simulink model "may14bdrc"  (R2015a)
settings: Solver=ode4  StartTime=0.0  StopTime=inf  FixedStep=BKIN_STEP_TIME  RelTol=1e-3
StartFcn:
  |  warndlg('Dexterit-E models cannot run under simulation. Please compile your model and run it from within Dexterit-E.');set_param(bdroot,'SimulationCommand','stop')
model workspace (MAT data in the model file):
  BARRIER_ROW = 5
  BKIN_KINEMATIC_FRAME_SIZE = 400
  BKIN_STEP_TIME = 0.00025
  CIRCLE_ROW = 2
  CIRCLE_STROKE = 10
  CIRCLE_STROKE_W = 11
  E_BARRIER_HIT = 6
  E_COLLISION_HIT = 7
  E_ENTER_PRESHOT_AREA = 2
  E_ENTER_START_AREA = 12
  E_EXIT = 13
  E_EXIT_PRESHOT_AREA = 10
  E_GOAL_HIT = 8
  E_GOAL_REACHED = 5
  E_NO_EVENT = 0
  E_PRESHOT_ROW = 4
  E_TARGET_OUT_OF_BOUNDS = 9
  E_TRIAL_BEGIN = 1
  E_TRIAL_ENDED = 3
  FIRST_STATE_FILL = 9
  FORCE_MULTIPLIER = 1
  F_BUMP = 1
  GOAL_ROW = 8
  GOAL_TIME = 15
  HEIGHT = 6
  INVISIBLE_FILL = 15
  LOAD_ROW = 4
  MASS_BARRIER = 6
  MASS_CIRCLE = 2
  MASS_RECT = 3
  NEW_FLOAT = 10
  NEW_ROW = 9
  NEW_TEXTSIZE = 11
  PERT_DUR = 5
  PERT_RAMP = 4
  PRESHOT_ROW = 7
  RADIUS_LOG = 4
  RADIUS_VIS = 5
  RECT_FILL = 12
  RECT_ROW = 3
  RECT_STROKE = 13
  RECT_STROKE_W = 14
  ROTATION = 7
  SECONDS = 1
  SECOND_STATE_FILL = 8
  SHOT_READY_TIME = 13
  SHOT_SET_TIME = 14
  START_HOLD_TIME = 12
  START_ROW = 6
  TRIAL_FAILURE = 11
  WIDTH = 3
  col_x = 1
  col_y = 2
undefined symbols (not defined in the file): slselsubs
libraries: Video x7, General x3, KINARM_loads x2, KINARM_EP_loads x1, KINARM_general x1, simulink x1, slrtlib x1
(part 2 of 3)

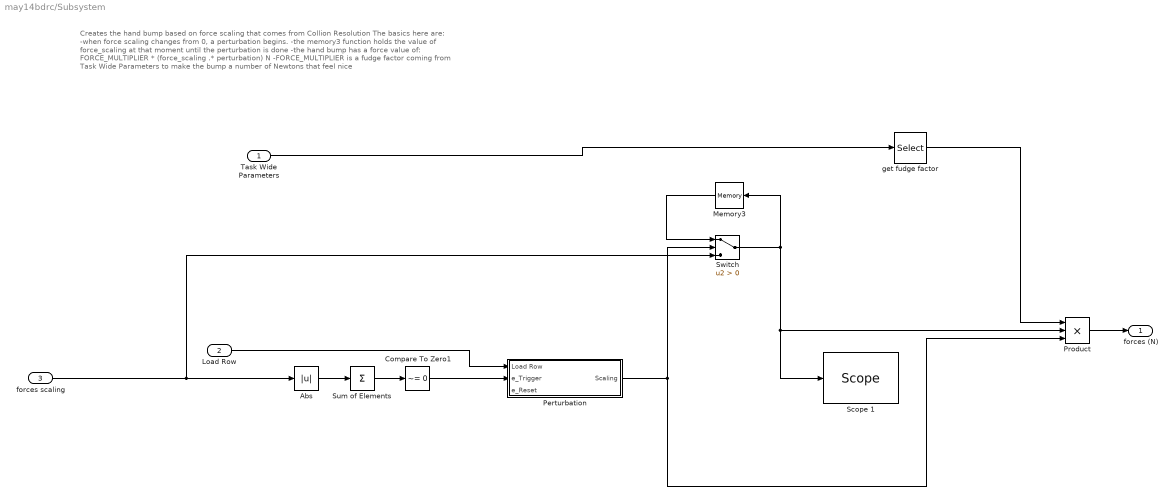
== system may14bdrc/Subsystem ==
  note: Creates the hand bump based on force scaling that comes from Collion Resolution
      |
      | The basics here are:
      | -when force scaling changes from 0, a perturbation begins.
      | -the memory3 function holds the value of force_scaling at that moment until the perturbation is done
      | -the hand bump has a force value of: FORCE_MULTIPLIER * (force_scaling .* perturbation) N
      | -FORCE_MULTIPLIER is a fudge factor coming from Task Wide Parameters to make the bump a number of Newtons that feel nice
  Task Wide Parameters : Inport
  Load Row : Inport  Port=2
  forces scaling : Inport  Port=3
  Abs : Abs
  Compare To Zero1 : simulink/Logic and Bit Operations/Compare To Zero  relop=~=  OutDataTypeStr=uint8  ZeroCross=off
  Memory3 : Memory  InheritSampleTime=on
  Perturbation : Subsystem  AncestorBlock=KINARM_loads/Perturbation  mask(Perturbation){loadcol=[PERT_RAMP PERT_DUR PERT_RAMP]}
      mask prompts: loadcol "Load Table Columns [colA colB colC]"
      mask help:
      | The Perturbation block creates a time-varying output that is used to ‘window’ the output of other load  blocks.  For example, to create a force pulse, the 'scaling' output of this block would be wired into the 'scaling' input of the Constant_Loads_(hand) block.
      |
      | The shape of the scaling window is trapezoidal and composed of three sections:
      |
      | 1. A linear on-ramp where the scaling output goes from 0 to 1. The duration of this ramping is determined from the value in column A.
      | 2. A duration where the scaling output is 1 (i.e. maximal). This duration is determined from the value in column B.
      | 3. A linear off-ramp where the scaling output goes from 1 to 0. The duration of this ramping is determined from the value in column C.
      |
      | (Note: scaling output = 0 between perturbations)
      |
      | The values in columns A, B & C must all be in milliseconds.
      |
      | The reset input is used to immediately stop the perturbation and set the output scaling to zero. The reset input does not need to be called between uses.
      mask init:
      | library = 'KINARM_loads';
      | numCol = 3;
      | [inputname1, inputname2, inputname3, outputname, columntext] = loadBlockInitCommands(gcb, library, numCol);
      mask Help:
      | Used to create a perturbation 'window' for scaling other load blocks.
      | 
      | <H2>Library </H2>
      | KINARM EXO loads
      | 
      | <H2>Description </H2>
      | The Perturbation block creates a time-varying output that is used to ‘window’ the output of other load blocks.  The 'scaling' output of the Perturbation block is typically wired to the 'scaling' input of another load block (note: the 'scaling' input of other loads blocks is hidden by default and must be shown by setting the 'Source for scaling' to 'external' within that block’s dialog box).
      | <P>
      | <P>
      | The perturbation window is started by sending a Stateflow event to the trigger input.  Once the perturbation has started, it continues in a deterministic fashion to its end unless a Stateflow event is sent to the 'reset' input, in which case the perturbation is canceled and the 'scaling' output is set to 0.
      | 
      | <p>The shape of the scaling window is trapezoidal and composed of three sections:
      | 
      | <ol>
      | <li>A linear on-ramp where the scaling output goes from 0 to 1. The duration of this ramping is determined from the value in column A.</li>
      | <li>A duration where the scaling output is 1 (i.e. maximal). This duration is determined from the value in column B.</li>
      | <li>A linear off-ramp where the scaling output goes from 1 to 0. The duration of this ramping is determined from the value in column C.</li>
      | </ol>
      | 
      | The ramp duration parameters [A, B, C] are found in the Load Table using the 'row' input to this block and the 'columns' parameter found in the dialog box for this block.
      | <p>For example, if the "row" input = 2, and "Load Table columns" are specified as [1 2 3], then using the sample Load Table below, the duration of the on ramp is 100 ms, constant torque is 200 ms, and the off ramp is 500 ms.
      | <br>
      | (Note: scaling output = 0 between perturbations)
      | 
      | <table border="1" cellpadding="5">
      | <tr><td></td><td>Ramp On</td><td>Const</td><td>Ramp off</td></tr>
      | <tr><td>Load 1</td><td>25</td><td>25</td><td>25</td></tr>
      | <tr><td>Load 2</td><td>100</td><td>200</td><td>500</td></tr>
      | <tr><td>Load 3</td><td>25</td><td>50</td><td>75</td></tr>
      | </table>
      | <P>
      | <B>row: </B> this scalar input indicates which row in the Load Table the ramp duration parameters [A, B, C] will come from.
      | <P>
      | <B>trigger: </B> this Stateflow event input starts the perturbation (triggered on either rising or falling; the Stateflow output event providing this trigger should have its Trigger setting set to ‘either’).  This input will be ignored if the Perturbation block is presently executing a perturbation.
      | <P>
      | <B>reset: </B> this Stateflow event input resets the perturbation (triggered on either rising or falling).  The reset will act immediately and force the Scaling output =0. This does not need to be called between used of the block. If you do not need to stop a perturbation prematurely, then this input can remain unconnected.
      | <P>
      | <B>scaling: </B> this scalar output is the time-dependent window created by this block.  Typically it is wired to the 'scaling' input of another load block.  It ranges in value from 0 to 1.
      | 
      | <H2>Parameters and Dialog Box</H2>
      | <B>Load Table Columns:</B> a 3x1 vector with the elements corresponding to the columns in the Load Table for parameters A, B and C.  If a parameter is not going to be in the Load Table, then the value 0 should be used in the "Load Table Columns" vector (e.g. if there is to be no on-ramp or off-ramp, and the peak-duration coefficients is in column 2, then the "Load Table Columns" vector should be [0 2 0], which indicates that A and C are not specified in the Load Table and so they are set =0).  The same column may be used for more than one parameter, so if the on-ramp and off-ramp are to be equal, then the same column can be specified twice (e.g. [1 2 1]).
      | <P>
      |  All durations are specified in milliseconds.
      | 
      | <H2>Examples</H2>
      | <B>Example 1. </B> Suppose we wish to create a torque pulse with no on or off ramp and a peak duration specified in column 3 of the Load Table.  The 'scaling' output of the Perturbation block would be wired to the 'scaling' input of the Constant_Loads_(joints) block (after setting 'Source for scaling' to 'external' within the Constant_Loads_(joints) block).  The Load Table Columns setting in the dialog box for the Perturbation block would be set to [0 3 0], which indicates no on-ramp or off-ramp and that the peak duration will be in column 3 of the Load Table.
      | <P>
      | <B>Example 2. </B> Suppose we wish to create a force pulse at the hand with an on-ramp and off-ramp of the same duration (specified in column3 of the Load Table) and a peak duration specified in column 4 of the Load Table.  The 'scaling' output of the Perturbation block would be wired to the 'scaling' input of the Constant_Loads_(hand) block (after setting 'Source for scaling' to 'external' within the Constant_Loads_(hand) block).  The Load Table Columns setting in the dialog box for the Perturbation block would be set to [3 4 3], which indicates that the on-ramp and off-ramp durations are specified in column 3 of the Load Table and that the peak duration will be in column 4 of the Load Table.
      | 
      | <H2>Related Blocks </H2>
      | KINARM_Exo_Apply_Loads<BR>
      | Constant_Loads_(hand)<BR>
      | Constant_Loads_(joint)
      mask Callback loadcol:
      | %%%%
      | % Because of bugs iN R2007, R2010a and R2013a (which have been reported to Mathworks), the following code
      | % is required here because in the Initialization Section it will ONLY correctly update those Mask Parameters that are hidden
      | % when the OK button is clicked (NOTE: the initialization code will correctly update all Mask Parameters when the Apply button
      | % is clicked, the bug is that it should also update everything when the OK button is clicked in the absence of an Apply click)
      | %
      | % Adding a set_param call which updates one of the mask parameters will call the initialization code to run, which "avoids"
      | % this bug. This code should be removed once Mathworks has fixed this bug.
      | 
      | temp = get_param(gcb, 'loadcol');
      | set_param(gcb, 'loadcol', temp);
      mask Display:
      | disp(columntext);
      | port_label('output',1,outputname);
      | port_label('input',1, inputname1);
      | port_label('input',2, inputname2);
      | port_label('input',3, inputname3);
  Product : Product  Inputs=3
  Scope 1 : slrtlib/Displays and Logging/Scope   scopeno=4  scopetype=Target  autostart=off  viewmode=Graphical redraw  formatstr='%15.6f'  grid=on  ylimits=[0,0]  nosamples=250  noprepostsamples=0  interleave=1  triggermode=FreeRun  triggersignal=1  trigsignalfromport=off  triggerlevel=0.0  triggerslope=Either  triggerscope=1  triggersample=0  filename=data.dat  mode=Lazy  writesize=512  autorestart=off  dynamicfilemode=off  maxwritefilesize=512*1024^2
  Sum of Elements : Sum  Inputs=+
  Switch : Switch  Criteria=u2 > Threshold
  get fudge factor : Selector  IndexOptions=Index vector (dialog)  Indices=FORCE_MULTIPLIER  OutputSizes=1
  forces (N) : Outport
  wires:
  Compare To Zero1/1 -> Perturbation/2(e_Trigger)
  Sum of Elements/1 -> Compare To Zero1/1
  forces scaling/1 -> Switch/3, Abs/1
  get fudge factor/1 -> Product/1
  Switch/1 -> Memory3/1, Scope 1/1, Product/2
  Perturbation/1(Scaling) -> Product/3, Switch/2
  Abs/1 -> Sum of Elements/1
  Memory3/1 -> Switch/1
  Load Row/1 -> Perturbation/1(Load Row)
  Product/1 -> forces (N)/1
  Task Wide Parameters/1 -> get fudge factor/1

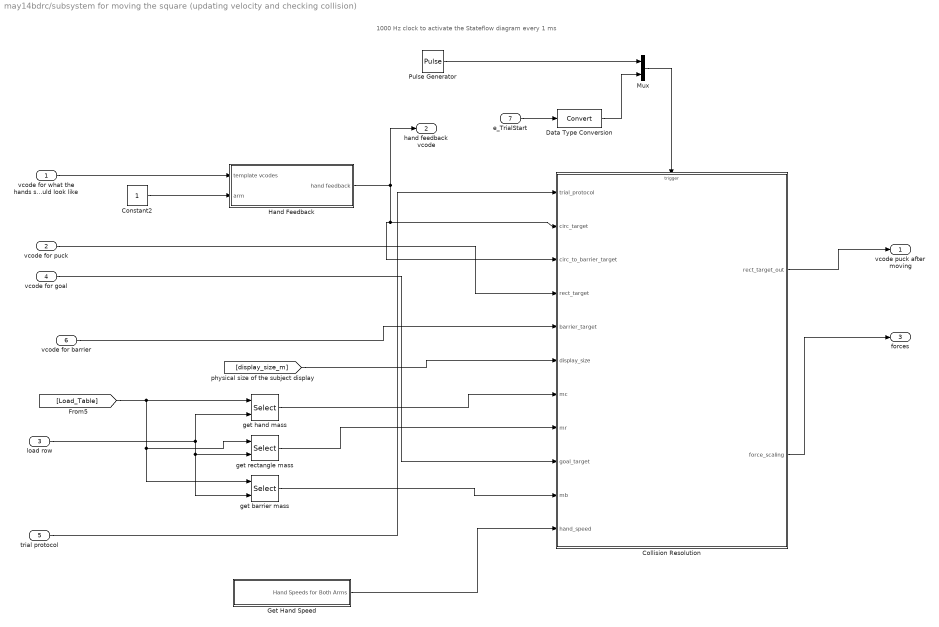
== system may14bdrc/subsystem for moving the square (updating velocity and checking collision) ==
  note: 1000 Hz clock to activate the Stateflow diagram every 1 ms
  vcode for what the hands should look like : Inport  PortDimensions=[1 70]
  vcode for puck : Inport  Port=2  PortDimensions=[1 70]  LockScale=on
  load row : Inport  Port=3
  vcode for goal : Inport  Port=4  PortDimensions=[1 70]
  trial protocol : Inport  Port=5
  vcode for barrier : Inport  Port=6  PortDimensions=[1 70]
  e_TrialStart : Inport  Port=7
  Collision Resolution : Stateflow chart  TreatAsAtomicUnit=on
      settings: PermitHierarchicalResolution=ParametersOnly
  Constant2 : Constant
  Data Type Conversion : DataTypeConversion
  Get Hand Speed : Subsystem
  Hand Feedback : Subsystem
  Mux : Mux  Inputs=2
  Pulse Generator : DiscretePulseGenerator  PulseType=Time based  Period=1/1000  PulseWidth=50
  get barrier mass : Selector  NumberOfDimensions=2  IndexOptions=Index vector (port),Index vector (dialog)  Indices=MASS_RECT,MASS_RECT  OutputSizes=1,1
  get hand mass : Selector  NumberOfDimensions=2  IndexOptions=Index vector (port),Index vector (dialog)  Indices=MASS_CIRCLE,MASS_CIRCLE  OutputSizes=1,1
  get rectangle mass : Selector  NumberOfDimensions=2  IndexOptions=Index vector (port),Index vector (dialog)  Indices=MASS_RECT,MASS_RECT  OutputSizes=1,1
  vcode puck after moving : Outport
  hand feedback vcode : Outport  Port=2
  forces : Outport  Port=3
  wires:
  load row/1 -> get barrier mass/2, get rectangle mass/2, get hand mass/2
  Hand Feedback/1(hand feedback) -> hand feedback vcode/1, Collision Resolution/3(circ_to_barrier_target), Collision Resolution/2(circ_target)
  Collision Resolution/1(rect_target_out) -> vcode puck after moving/1
  vcode for puck/1 -> Collision Resolution/4(rect_target)
  Get Hand Speed/1(Hand Speeds for Both Arms) -> Collision Resolution/11(hand_speed)
  get hand mass/1 -> Collision Resolution/7(mc)
  get rectangle mass/1 -> Collision Resolution/8(mr)
  Pulse Generator/1 -> Mux/1
  [display_size_m] -> Collision Resolution/6(display_size)
  Collision Resolution/2(force_scaling) -> forces/1
  vcode for what the hands should look like/1 -> Hand Feedback/1(template vcodes)
  Constant2/1 -> Hand Feedback/2(arm)
  vcode for goal/1 -> Collision Resolution/9(goal_target)
  trial protocol/1 -> Collision Resolution/1(trial_protocol)
  vcode for barrier/1 -> Collision Resolution/5(barrier_target)
  [Load_Table] -> get barrier mass/1, get rectangle mass/1, get hand mass/1
  get barrier mass/1 -> Collision Resolution/10(mb)
  Mux/1 -> Collision Resolution/Trigger
  e_TrialStart/1 -> Data Type Conversion/1
  Data Type Conversion/1 -> Mux/2

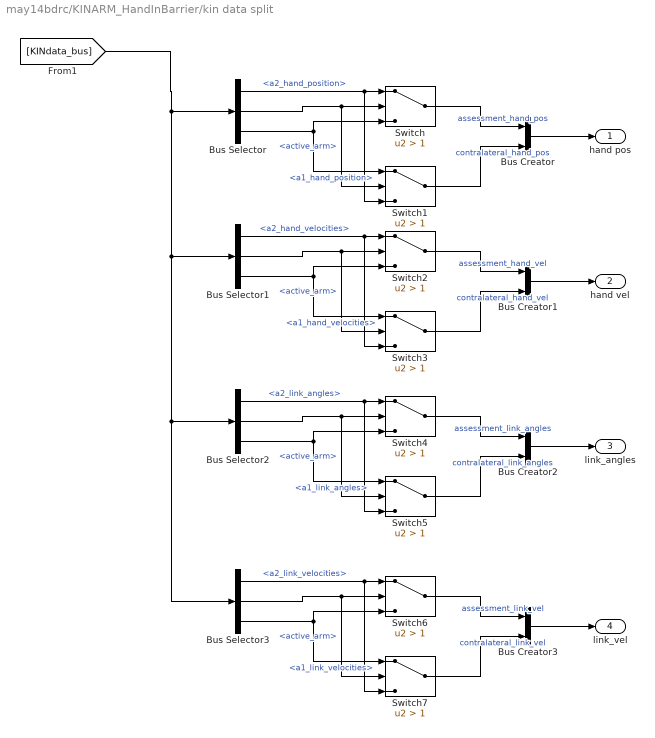
== system may14bdrc/KINARM_HandInBarrier/kin data split ==
  Bus Creator{,1..3} (4 alike) : BusCreator  Inputs=2
  Bus Selector : BusSelector  OutputSignals=Robot2.a2_hand_position,KINDataGeneral.active_arm,Robot1.a1_hand_position
  Bus Selector1 : BusSelector  OutputSignals=Robot2.a2_hand_velocities,KINDataGeneral.active_arm,Robot1.a1_hand_velocities
  Bus Selector2 : BusSelector  OutputSignals=Robot2.a2_link_angles,KINDataGeneral.active_arm,Robot1.a1_link_angles
  Bus Selector3 : BusSelector  OutputSignals=Robot2.a2_link_velocities,KINDataGeneral.active_arm,Robot1.a1_link_velocities
  Switch{,1..7} (8 alike) : Switch  Criteria=u2 > Threshold  Threshold=1
  hand pos : Outport
  hand vel : Outport  Port=2
  link_angles : Outport  Port=3
  link_vel : Outport  Port=4
  wires:
  Bus Selector/1 -> Switch1/3, Switch/1  "<a2_hand_position>"
  Switch/1 -> Bus Creator/1  "assessment_hand_pos"
  Switch1/1 -> Bus Creator/2  "contralateral_hand_pos"
  Bus Creator/1 -> hand pos/1
  Bus Selector/3 -> Switch1/1, Switch/3  "<a1_hand_position>"
  Bus Selector/2 -> Switch1/2, Switch/2  "<active_arm>"
  Bus Selector1/1 -> Switch3/3, Switch2/1  "<a2_hand_velocities>"
  Switch2/1 -> Bus Creator1/1  "assessment_hand_vel"
  Switch3/1 -> Bus Creator1/2  "contralateral_hand_vel"
  Bus Creator1/1 -> hand vel/1
  Bus Selector1/3 -> Switch3/1, Switch2/3  "<a1_hand_velocities>"
  Bus Selector1/2 -> Switch3/2, Switch2/2  "<active_arm>"
  Bus Selector2/1 -> Switch5/3, Switch4/1  "<a2_link_angles>"
  Switch4/1 -> Bus Creator2/1  "assessment_link_angles"
  Switch5/1 -> Bus Creator2/2  "contralateral_link_angles"
  Bus Creator2/1 -> link_angles/1
  Bus Selector2/3 -> Switch5/1, Switch4/3  "<a1_link_angles>"
  Bus Selector2/2 -> Switch5/2, Switch4/2  "<active_arm>"
  Bus Selector3/1 -> Switch7/3, Switch6/1  "<a2_link_velocities>"
  Switch6/1 -> Bus Creator3/1  "assessment_link_vel"
  Switch7/1 -> Bus Creator3/2  "contralateral_link_vel"
  Bus Creator3/1 -> link_vel/1
  [KINdata_bus] -> Bus Selector3/1, Bus Selector2/1, Bus Selector1/1, Bus Selector/1
  Bus Selector3/3 -> Switch7/1, Switch6/3  "<a1_link_velocities>"
  Bus Selector3/2 -> Switch7/2, Switch6/2  "<active_arm>"

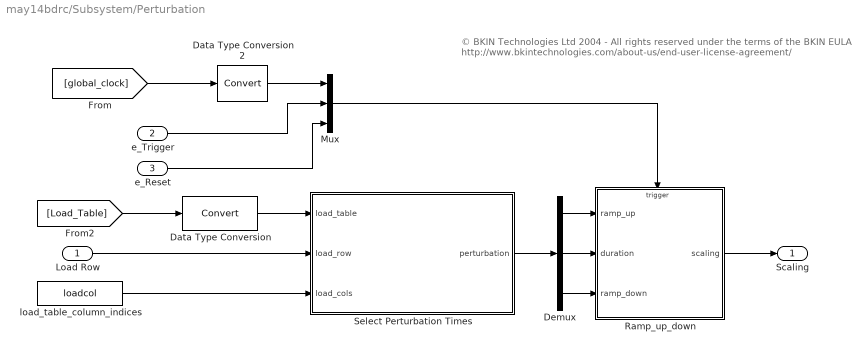
== system may14bdrc/Subsystem/Perturbation ==
  note: © BKIN Technologies Ltd 2004  - All rights reserved under the terms of the BKIN EULA
      | http://www.bkintechnologies.com/about-us/end-user-license-agreement/
  Load Row : Inport
  e_Trigger : Inport  Port=2
  e_Reset : Inport  Port=3
  Data Type Conversion : DataTypeConversion
  Data Type Conversion2 : DataTypeConversion
  Demux : Demux  Outputs=3
  Mux : Mux  Inputs=3
  Ramp_up_down : Stateflow chart  TreatAsAtomicUnit=on
      settings: PermitHierarchicalResolution=ParametersOnly
  Select Perturbation Times : MATLAB Function  TreatAsAtomicUnit=on
      settings: PermitHierarchicalResolution=ParametersOnly
  load_table_column_indices : Constant  Value=loadcol
  Scaling : Outport
  wires:
  Data Type Conversion2/1 -> Mux/1
  Mux/1 -> Ramp_up_down/Trigger
  Demux/3 -> Ramp_up_down/3(ramp_down)
  Demux/2 -> Ramp_up_down/2(duration)
  Demux/1 -> Ramp_up_down/1(ramp_up)
  [global_clock] -> Data Type Conversion2/1
  Ramp_up_down/1(scaling) -> Scaling/1
  e_Trigger/1 -> Mux/2
  e_Reset/1 -> Mux/3
  [Load_Table] -> Data Type Conversion/1
  Load Row/1 -> Select Perturbation Times/2(load_row)
  load_table_column_indices/1 -> Select Perturbation Times/3(load_cols)
  Select Perturbation Times/1(perturbation) -> Demux/1
  Data Type Conversion/1 -> Select Perturbation Times/1(load_table)

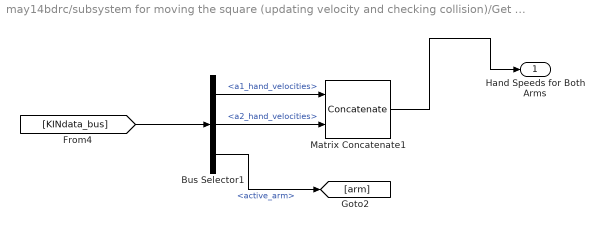
== system may14bdrc/subsystem for moving the square (updating velocity and checking collision)/Get Hand Speed ==
  Bus Selector1 : BusSelector  OutputSignals=Robot1.a1_hand_velocities,Robot2.a2_hand_velocities,KINDataGeneral.active_arm
  Matrix Concatenate1 : Concatenate  Mode=Multidimensional array
  Hand Speeds for Both Arms : Outport
  wires:
  [KINdata_bus] -> Bus Selector1/1
  Bus Selector1/1 -> Matrix Concatenate1/1  "<a1_hand_velocities>"
  Matrix Concatenate1/1 -> Hand Speeds for Both Arms/1
  Bus Selector1/2 -> Matrix Concatenate1/2  "<a2_hand_velocities>"
  Bus Selector1/3 -> [arm]  "<active_arm>"

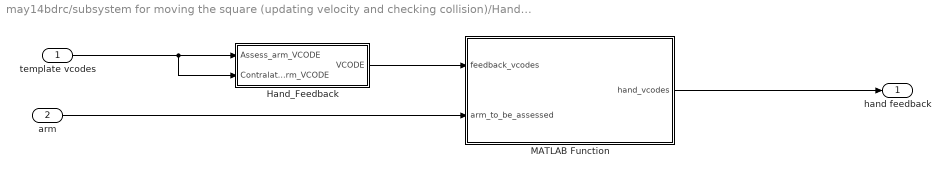
== system may14bdrc/subsystem for moving the square (updating velocity and checking collision)/Hand Feedback ==
  template vcodes : Inport
  arm : Inport  Port=2
  Hand_Feedback : Subsystem  AncestorBlock=KINARM_general/Hand_Feedback  mask(Hand_Feedback){feedback_cntl_src=style and status}
      mask prompts: feedback_cntl_src "Task Program control of style and status"
      mask help:
      | This block controls various options for hand feedback (i.e. fingertip position)  to be shown to the subject.
      |
      | Task Program control of style and status refers to whether the Program Task will explicity control the style and/or status of the hand feedback.
      mask init:
      | block_path = gcb;  % store block path, as gcb may change with block operations
      | 
      | %%% Handle background colours if link status changes.  
      | checkBackgroundColour(block_path, 'KINARM_general');
      | 
      | 
      | feedback_cntl_source=get_param(gcb,'feedback_cntl_src');
      | 
      | if feedback_cntl_source(1:4)=='none'
      |     block1type='Constant';
      |     block2type='Constant';
      |     block3type='Constant';
      | elseif feedback_cntl_source(1:4)=='stat'
      |     block1type='Constant';
      |     block2type='Constant';
      |     block3type='Inport';
      | else 
      |     block1type='Inport';
      |     block2type='Inport';
      |     block3type='Constant';
      | end
      | 
      | hasOldName1 = ~isempty(find_system(gcb, 'FollowLinks', 'on', 'LookUnderMasks', 'all', 'name', 'Dom_VCODE'));
      | hasOldName2 = ~isempty(find_system(gcb, 'FollowLinks', 'on', 'LookUnderMasks', 'all', 'name', 'non-Dom_VCODE'));
      | 
      | block1name='Assess_arm_VCODE';
      | block2name='Contralateral_arm_VCODE';
      | block1path=[gcb '/' block1name];
      | block2path=[gcb '/' block2name];
      | 
      | if hasOldName1
      | 	set_param([gcb '/Dom_VCODE'],'name', block1name);
      | end
      | 
      | if hasOldName2
      | 	set_param([gcb '/non-Dom_VCODE'],'name', block2name);
      | end
      | 
      | if ~strcmp(get_param(block1path,'blocktype'),block1type)
      | 	pos=get_param(block1path,'position');
      | 	delete_line(gcb, [block1name '/1'], 'Reshape/1');
      | 	delete_block(block1path);
      | 	add_block(['built-in/' block1type], block1path,'Name',block1name);
      | 	set_param(block1path,'position',pos);
      | 	add_line(gcb, [block1name '/1'], 'Reshape/1');
      | end
      | 
      | if ~strcmp(get_param(block2path,'blocktype'),block2type)
      | 	pos=get_param(block2path,'position');
      | 	delete_line(gcb, [block2name '/1'], 'Reshape1/1');
      | 	delete_block(block2path);
      | 	add_block(['built-in/' block2type],block2path,'Name',block2name);
      | 	set_param(block2path,'position',pos);
      | 	add_line(gcb, [block2name '/1'], 'Reshape1/1');
      | end
      | 
      | block3name='feedback_status';
      | block3path=[gcb '/' block3name];
      | if ~strcmp(get_param(block3path,'blocktype'),block3type)
      | 	pos=get_param(block3path,'position');
      | 	delete_line(gcb, [block3name '/1'], 'FeedFwdArm/3');
      | 	delete_block(block3path);
      | 	add_block(['built-in/' block3type],block3path,'Name',block3name);
      | 	set_param(block3path,'position',pos);
      | 	add_line(gcb, [block3name '/1'], 'FeedFwdArm/3');
      | end
      | 
      | if feedback_cntl_source(1:4)=='none'
      | 	set_param(block1path,'Value','[1:70]');
      | 	set_param(block2path,'Value','[71:140]');
      | elseif feedback_cntl_source(1:4)=='stat'
      | 	set_param(block1path,'Value','[1:70]');
      | 	set_param(block2path,'Value','[71:140]');
      | end
      mask Help:
      | Creates VCODE for drawing hand position (fingertip).
      | <P>
      | <H2>Library </H2>
      | KINARM general
      | 
      | <H2>Description </H2>
      | This block controls various options for drawing hand feedback.  (Note: although it is called hand feedback, it is actually the fingertip position that is shown).  Three options are available (as chosen in the Parameters and Dialog box):
      | <P>
      | (i) GUI control of feedback style and status
      | <Blockquote>
      | No inputs are required for this option.  The Task Program has no control over the style or status of the hand feedback.
      | </Blockquote>
      | (ii) Task Program control of feedback status and GUI control of style
      | <Blockquote>
      | If Task Program control of feedback status is chosen, then one input appears for this block:<P>
      | <B> feedback_status: </B> this scalar input dynamically controls the status of the hand feedback as per the following:
      | <P>
      | 0 = (no hand feedback)<BR>
      | 1 = ("arm to be assessed" hand feedback only)<BR>
      | 2 = (contralateral arm hand feedback only)<BR>
      | 3 = (hand feedback on for both hands)<BR>
      | </Blockquote>
      | (iii) Task Program control of both feedback style and status.
      | <Blockquote>
      | 
      | If Task Program control of feedback status and style is chosen, then two inputs appear for this block:<P>
      | <B> Assess_arm_VCODE: </B>  this vector input dynamically controls the status and style of the hand feedback for the "arm to be assessed" the operator selected in Dexterit-E.
      | <P>
      | <B> Contralateral_arm_VCODE:</B>  this vector input dynamically controls the status and style of the hand feedback for the contralateral hand.
      | <P>
      | For both the Assess_arm_VCODE and the Contralateral_arm_VCODE, the input vectors must be in the appropriate VCODE format (for more information on the details of a VCODE, please right click on the Show_Target block in the video library, "Look Under Mask" and open the Embedded Matlab function).  Note that the position information in the Dom_VCODE and non-Dom_VCODE are overwritten in this block, but all other aspects of the VCODE are passed through to the output.
      | </Blockquote>
      | Note that if Task Program control is chosen for either hand feedback status or style, the GUI will still override these settings if the Task Protocol specifies that it should do so.
      | <P>
      | There is one output from this block:
      | <P>
      | <B> VCODE: </B> this output is 2-row matrix containing 2 VCODEs.  The first VCODE is for the dominant hand feedback and the second VCODE is for the non-dominant hand feedback.  This output must go to the Process_Video_CMD block of the video library for the hand feedback to actually be shown (if any other visual targets are to be displayed, then this VCODE output must be concatenated with the other VCODES prior to connection to the Process_Video_CMD block - see Help for the Process_Video_CMD block for more information).
      | <H2>Parameters and Dialog Box</H2>
      | <B>Task Program control of style and status</B> refers to whether the Program Task will explicity control the style and/or status of the hand feedback.  The three options are: none, status only, or status and style.
      | <P>
      |  - Choosing none means that style and status are always controlled by the GUI.
      | <P>
      |  - Choosing status only means that the GUI always controls the hand feedback style, but also will create an input to this block allowing the end user to control the status dynamically.  Allowable input values are: 0 (no hand feedback), 1 (dominant hand feedback only), 2 (non-dominant hand feedback only) or 3 (hand feedback on for both hands)
      |  <P>
      | - Choosing status and style means that both the hand feedback status and style can be controlled dynamically by the Task Program.  If this option is selected, then two inputs will be created for this block: dominant VCODE and non-dominant VCODE.  These two inputs require a proper VCODE (e.g. from a Show_Target block) for each.  Because status and style are both part of a VCODE, there is no separate input for hand feedback status.  Note: any position information of these input VCODEs is overwritten by this block by the appropriate fingertip locations.
      | <P>
      | 
      | <H2>Related Blocks </H2>
      | DataLogging<BR>
      | Show_Target<BR>
      | Process_Video_CMD
      mask TypeOptions feedback_cntl_src: none | status only | style and status
  MATLAB Function : MATLAB Function  TreatAsAtomicUnit=on
      settings: PermitHierarchicalResolution=ParametersOnly
  hand feedback : Outport
  wires:
  template vcodes/1 -> Hand_Feedback/2(Contralateral_arm_VCODE), Hand_Feedback/1(Assess_arm_VCODE)
  Hand_Feedback/1(VCODE) -> MATLAB Function/1(feedback_vcodes)
  arm/1 -> MATLAB Function/2(arm_to_be_assessed)
  MATLAB Function/1(hand_vcodes) -> hand feedback/1

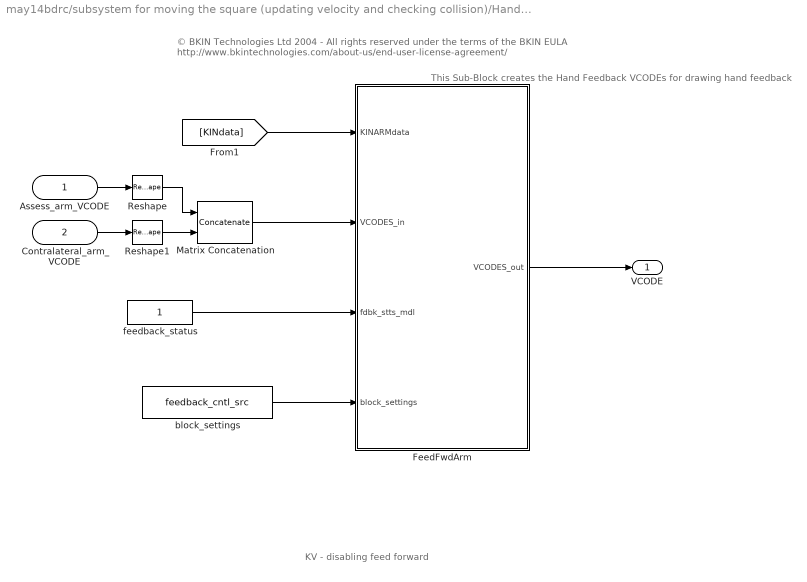
== system may14bdrc/subsystem for moving the square (updating velocity and checking collision)/Hand Feedback/Hand_Feedback ==
  note: KV - disabling feed forward
  note: This Sub-Block creates the Hand Feedback VCODEs for drawing hand feedback
  note: © BKIN Technologies Ltd 2004  - All rights reserved under the terms of the BKIN EULA
      | http://www.bkintechnologies.com/about-us/end-user-license-agreement/
  Assess_arm_VCODE : Inport
  Contralateral_arm_VCODE : Inport  Port=2
  FeedFwdArm : MATLAB Function  TreatAsAtomicUnit=on
      settings: PermitHierarchicalResolution=ParametersOnly  RTWSystemCode=Nonreusable function  RTWFileNameOpts=Use function name
  Matrix Concatenation : Concatenate  Mode=Multidimensional array
  Reshape : Reshape  OutputDimensionality=Row vector (2-D)
  Reshape1 : Reshape  OutputDimensionality=Row vector (2-D)
  block_settings : Constant  Value=feedback_cntl_src
  feedback_status : Constant
  VCODE : Outport
  wires:
  feedback_status/1 -> FeedFwdArm/3(fdbk_stts_mdl)
  FeedFwdArm/1(VCODES_out) -> VCODE/1
  block_settings/1 -> FeedFwdArm/4(block_settings)
  Matrix Concatenation/1 -> FeedFwdArm/2(VCODES_in)
  [KINdata] -> FeedFwdArm/1(KINARMdata)
  Reshape1/1 -> Matrix Concatenation/2
  Reshape/1 -> Matrix Concatenation/1
  Assess_arm_VCODE/1 -> Reshape/1
  Contralateral_arm_VCODE/1 -> Reshape1/1

== stateflow chart may14bdrc/subsystem for moving the square (updating velocity and checking collision)/Collision Resolution ==
  settings: sampleTime=0.001
  state Initialize/
    % Stateflow starts here when task is loaded
    entry: force_scaling = [0 0 0 0];
    rect_target_out = zeros(1,70);
    rect_vel = [0 0];
    rect_offset_position = [0 0];
  state Moving_Targets_and_Colliding_Them
    %there are 4 parallel states here. They each execute in the same cycle but in a specific order (see top right of the state)
    % state 3 is the important one - it simply says "move the square according to its velocity"
    % states 1 and 2 check collisions to update that velocity before we get to state 3
    % state 4 then checks to see if we ended up outside the screen and if so, to take us back to the start position
    state CollisionWithHand/ [parallel]
      % this substate will handle collision checks between hands and the square
      settings: executionOrder=1
      state StartWithSpeed0/
        %
        entry:
        rect_vel = [0 0];
        rect_offset_position = [0 0];
      state WaitForCollision/
        entry,during: % state where we wait for collisions to happen
        force_scaling = [0 0 0 0];
        during:
        target_colliding = check_collision(circ_target, rect_target, rect_offset_position)
      state ResolveTargetCollision
        during: % if something collided, we're going to separate the two objects and then use elastic collision to update velocities
        % eject the rectangle
        rect_offset_position = eject( circ_target( target_colliding,:), rect_target, rect_offset_position);
        prev_vel = rect_vel;
        hand_vel = hand_speed( target_colliding,:)/1e3;
        % elastic collision equations - here m = 1 and is the same for hand and puck. It is used here to provide relative mass
        % between the two objects. The forces here will be further multiplied by a fudge factor (see the Simulink forces section)
        rect_vel = (mr - mc)/(mr + mc)*rect_vel + 2*mc/(mc + mr)*hand_vel;
        % hand_vector = [1 2; 3 4];
        hand_vector = [1 2];
        % a bump will be generated that will be proportional to change in velocity
        force_scaling(hand_vector(target_colliding,:)) = prev_vel - rect_vel;
      WaitForCollision -> StartWithSpeed0 [order 2] : e_Trial_Start
      StartWithSpeed0 -> WaitForCollision
      WaitForCollision -> ResolveTargetCollision [order 1] : [ target_colliding]
      ResolveTargetCollision -> WaitForCollision : [~check_collision(circ_target( target_colliding,:), rect_target, rect_offset_position)]
          | /{target_colliding=0}
    state UpdatePosition/ [parallel]
      during:
      rect_target_out = rect_target;
      rect_offset_position = rect_offset_position + rect_vel;
      rect_target_out(3:4) = rect_target_out(3:4)+rect_offset_position
      settings: executionOrder=2
  (default) -> Initialize
  Initialize -> StartWithSpeed0
  data: colliding_target function_output; cursor_vcode function_input; puck_vcode function_input; puck_offset function_input; ejected_puck_offset function_output; cursor_vcode function_input; puck_vcode function_input; puck_offset function_input; trial_protocol input; circ_target input double; circ_to_barrier_target input; rect_target_out output size=[1 70]; rect_target input; barrier_target input size=[1 70]; display_size input; force_scaling output; mc input; mr input; hand_vector local; rect_vel local; prev_vel local; target_colliding local; hand_vel local; rect_offset_position local double; goal_target input; mb input size=1; barrier_colliding local; hand_speed input; check_collision_barrier1 local; barrier_vel local; force_scaling_barrier local; rect_y local; rect_w local; rect_h local; rect_x local; goal_h local; goal_y local; goal_w local; goal_x local; rect_top local; goal_top local; hand_offset_position local; prev_hand_vel local; rect_left local; rect_bottom local; goal_right local; rect_right local; goal_bottom local; goal_left local; new_hand_posistion_c local
  events: e_clk input RISING_EDGE_EVENT; e_Trial_Start input EITHER_EDGE_EVENT
  function colliding_target = check_collision(cursor_vcode, puck_vcode, puck_offset):
    | function colliding_target = check_collision(cursor_vcode, puck_vcode, puck_offset)
    | 
    | % calculates collision between 2 circiular cursors (ie. either hand feedback) and
    | % puck (also a circle)
    | % inputs:
    | %        cursor_vcode - 2x70 matrix that is 2 circle vcodes (right hand is
    | %                       top row, left hand is bottom row
    | %        puck_vcode - 1x70 vector that is a puck vcode
    | %        puck_offset - 1x2 position offset vector for puck_vector_in to calculate
    | %                         where the puck is
    | % outputs:
    | %        colliding_target values:
    | %              0- if nothing colliding
    | %              1- if puck collided with right hand
    | %              2- if puck colliding with left hand
    | 
    | x_ind = 3;
    | y_ind = 4;
    | radius_ind = 10;
    | colliding_target = 0;
    | 
    | for ii = 1:1%size(cursor_vcode,1)
    | 	
    | 	current_cursor_vcode = cursor_vcode(ii,:);
    | 	
    | 	cursor_radius = current_cursor_vcode(radius_ind);
    | 	puck_radius = puck_vcode(radius_ind);
    | 	
    |     cursor_loc = current_cursor_vcode([x_ind y_ind]);
    |     puck_loc = puck_vcode([x_ind y_ind]) + puck_offset;
    | 	delta_loc = cursor_loc-puck_loc;
    | 	
    | 	intarget = (sqrt(sum(delta_loc.^2)) < (cursor_radius + puck_radius));
    | 	
    | 	%--------------%
    | 	
    | 	
    | 	if intarget
    | 		colliding_target = ii;
    | 		break;
    | 	end
    | 	
    | end
  function ejected_puck_offset = eject(cursor_vcode, puck_vcode, puck_offset):
    | function ejected_puck_offset = eject(cursor_vcode, puck_vcode, puck_offset)
    | 
    | % moves the puck_vcode out of a cursor_vcode if the two are
    | % overlapping
    | 
    | x_ind = 3;
    | y_ind= 4;
    | radius_ind = 10;
    | 
    | cursor_radius = cursor_vcode(radius_ind);
    | puck_radius = puck_vcode(radius_ind);
    | 
    | cursor_loc = cursor_vcode([x_ind y_ind]);
    | puck_loc = puck_vcode([x_ind y_ind]) + puck_offset;
    | delta_loc = puck_loc-cursor_loc;
    | 
    | current_puck_distance = sqrt(sum(delta_loc.^2));
    | ejected_puck_distance = cursor_radius+puck_radius;
    | 
    | ejected_delta_loc = delta_loc/current_puck_distance * ejected_puck_distance;
    | ejected_puck_loc = cursor_loc + ejected_delta_loc;
    | 
    | ejected_puck_offset = ejected_puck_loc - puck_vcode([x_ind y_ind]);
    | % ejected_puck_offset + puck_vcode([x_ind y_ind]) = cursor_loc + (puck_loc-cursor_loc)/sqrt(sum(puck_loc-cursor_loc.^2)) * (cursor_radius+puck_radius);

== matlab function may14bdrc/subsystem for moving the square (updating velocity and checking collision)/Hand Feedback/MATLAB Function ==
  data: feedback_vcodes input; arm_to_be_assessed input; hand_vcodes output
function hand_vcodes = fcn(feedback_vcodes, arm_to_be_assessed)
% the hand feedback vcodes are sorted like this:
%    <arm to be assessed vcode>
%    <contralateral arm> 
% but using this function I am going to sort the vcodes like this:
%    <right arm>
%    <left arm>
% because that will make it easier to track velocities and forces

if arm_to_be_assessed == 1
	hand_vcodes = feedback_vcodes;
else
	hand_vcodes = feedback_vcodes([2 1], :);
	%hand_vcodes = feedback_vcodes;
end

== stateflow chart may14bdrc/Trial_Control ==
  settings: sampleTime=0.001
  state Initialize/
    % Set variables
    entry:
    logging_enable = true;
    start_target_row = Trial_Protocol(START_ROW);
    preshot_area_row = Trial_Protocol(PRESHOT_ROW);
    cursor_row = Trial_Protocol(CIRCLE_ROW);
    puck_row = Trial_Protocol(RECT_ROW);
    barrier_target_row = Trial_Protocol(BARRIER_ROW);
    goal_target_row = Trial_Protocol(GOAL_ROW);
    load_row = Trial_Protocol(LOAD_ROW);
    trial_duration = Trial_Protocol(SECONDS);
    start_hold_time = Trial_Protocol(START_HOLD_TIME);
    shot_ready_time = Trial_Protocol(SHOT_READY_TIME);
    shot_set_time = Trial_Protocol(SHOT_SET_TIME);
    goal_time = Trial_Protocol(GOAL_TIME);
  state Main_Trial/
    % Each trial task only initializes variables and then runs for Trial_Protocol(SECONDS) seconds before stopping
    state StartHold/
      entry:
      start_target_state = 3;
      preshot_area_state=0;
      puck_state=0;
      goal_target_state=0;
      barrier_target_state=0;
      event_code = E_ENTER_START_AREA;
    state PreshotStart/
      % send e_Trial_End event
      entry:
      preshot_area_state=3;
      puck_state=2;
      goal_target_state=2;
      barrier_target_state=2;
      e_Trial_Start;
      event_code = E_ENTER_PRESHOT_AREA;
    state StartOn/
      entry:
      start_target_state = 2;
      preshot_area_state = 0;
      cursor_state = 2;
      puck_state = 0;
      barrier_target_state = 0;
      goal_target_state = 0;
      event_code = E_TRIAL_BEGIN;
    state PreshotMove/
      % send e_Trial_End event
      entry:
    state ShotReady/
      % send e_Trial_End event
      entry:
      event_code = E_EXIT;
    state ShotSet/
      % send e_Trial_End event
      entry:
      preshot_area_state=0;
    state Success/
      % send e_Trial_End event
      entry:
      puck_state=0;
      goal_target_state=3
    state PuckInGoal/
      % send e_Trial_End event
      entry:
    state Shot/
      % send e_Trial_End event
      entry:
      start_target_state=0;
    state Fail/
      % send e_Trial_End event
      entry:
      start_target_state=0;
      preshot_area_state = 0;
      cursor_state = 2;
      puck_state = 0;
      barrier_target_state = 0;
      goal_target_state = 0;
    StartHold -> PreshotStart [order 2] : after(start_hold_time,sec)
    StartOn -> StartHold [order 1] : [HandInTarget(start_target_row,1)==1]
    StartHold -> StartOn [order 1] : [HandInTarget(start_target_row,1)==0]
    PreshotStart -> StartHold [order 1] : [HandInTarget(preshot_area_row,1)==0]
    PreshotStart -> PreshotMove [order 2] : [HandInTarget(start_target_row,1)==0]
    ShotSet -> StartOn [order 1] : [HandInTarget(start_target_row,1)==0]
    PreshotMove -> StartOn [order 2] : [HandInTarget(preshot_area_row,1)==0]
    ShotReady -> PreshotMove [order 1] : [HandInTarget(start_target_row,1)==0]
    PreshotMove -> ShotReady [order 1] : [HandInTarget(start_target_row,1)==1]
    ShotReady -> ShotSet [order 2] : after(shot_ready_time,sec)
    ShotSet -> Shot [order 2] : after(shot_set_time,sec)
    Shot -> Fail [order 4] : [(PuckInBarrier(barrier_target_row,1)==1) || PuckInDisplay==0]
    PuckInGoal -> Success [order 1] : after(goal_time,sec)
    Shot -> PuckInGoal [order 3] : [PuckInTarget(goal_target_row,1)==1]
    PuckInGoal -> Fail [order 2] : [PuckInTarget(goal_target_row,1)==0]
    Shot -> Fail [order 2] : [HandInBarrier(barrier_target_row,1)==1]
    Shot -> Fail [order 1] : after(trial_duration,sec)
  state Inter_Trial_State/
    % send e_Trial_End event
    entry:
    e_Trial_End;
    event_code = E_TRIAL_ENDED;
  (default) -> Initialize
  Initialize -> StartOn
  Inter_Trial_State -> StartOn : after(1, sec)
  StartOn -> Inter_Trial_State [order 2] : after(trial_duration, sec)
  Main_Trial -> Inter_Trial_State : e_ExitTrialNow
  Fail -> Inter_Trial_State : after(0.3,sec)
  Success -> Inter_Trial_State : after(0.3,sec)
  data: logging_enable output boolean; event_code output; cursor_row output; cursor_state output; puck_row output; puck_state output; load_row output; Trial_Protocol input; trial_duration local; barrier_target_row output; barrier_target_state output; start_target_row output; start_target_state output; goal_target_row output; goal_target_state output; HandInTarget input double; preshot_area_state output; preshot_area_row output; start_hold_time local; shot_set_time local; shot_ready_time local; HandInBarrier input double; PuckInTarget input; goal_time local; PuckInBarrier input; PuckInDisplay input
  events: e_clk input RISING_EDGE_EVENT; e_ExitTrialNow input EITHER_EDGE_EVENT; e_Trial_End output EITHER_EDGE_EVENT; e_Trial_Start output EITHER_EDGE_EVENT

== matlab function may14bdrc/subsystem for moving the square (updating velocity and checking collision)/Hand Feedback/Hand_Feedback/FeedFwdArm ==
  settings: fimath=|
      | fimath(...
      | 'RoundMode', 'floor',...
      | 'OverflowMode', 'wrap',...
      | 'ProductMode', 'KeepLSB', 'ProductWordLength', 32,...
      | 'SumMode', 'KeepLSB', 'SumWordLength', 32,...
      | 'CastBeforeSum', false)
  data: KINARMdata input; VCODES_in input; VCODES_out output; fdbk_stts_mdl input; block_settings input
function VCODES_out  = fcn(KINARMdata,VCODES_in,fdbk_stts_mdl, block_settings)
%
% This function creates the VCODEs for the hand position feedback for both
% hands.  Various options in the Mask of the Simulink block in which this
% embedded Matlab file sits, allow the user to specify how often
% the hand feedback is updated as well as the source of the style and status
% of the hand feedback.  
%
% block_settings is the value chosen by the user in the Mask for parent Simulink
% block.  Note: that even if the block is wired up to accept Task Program 
% control of hand feedback style and status, this embedded Matlab file allows
% the GUI to over-ride those settings.  However, if the GUI requests that
% the parent block use Task Program control for the style and/or status when
% it has not been programmed in, then this embedded Matlab file handles this
% appropriately and ignore the request for Task Program control.  
%
% block_settings=1 -- parent block does not have any Task Program control over style or status
% block_settings=2 -- parent block has Task Program control over status only
% block_settings=3 -- parent block has Task Program control over both style and status
%
% fdbk_stts_mdl (only potentially used if block_settings=2) 
% fdbk_stts_mdl=0 -- neither hand on
% fdbk_stts_mdl=1 -- dominant hand on
% fdbk_stts_mdl=2 -- non-dominant hand on
% fdbk_stts_mdl=3 -- both hands on
%
% VCODES (only potentially used if block_settings=3) 
% VCODES for dominant and non-dominant, input to parent block 


dominant_arm=KINARMdata(3,1);
feedfwd=KINARMdata(3,2);				%amount of feedforward extrapolation for hand position(s)
fdbk_stts_GUI=KINARMdata(3,3);			%status of hand feedback requested from GUI
fdbk_src_GUI=KINARMdata(3,4);			%source of hand feedback style requested from GUI
fdbk_clr_GUI=KINARMdata(3,5);			%colour of hand feedback required by GUI
fdbk_radius_GUI=KINARMdata(3,6);		%radius of hand feedback required by GUI


%----------------Feedback Style ----------------
% IF GUI asks for feedback style from Task Program (fdbk_src_GUI==0)
% AND if Task Program has been chosen to supply feedback style (block_settings==3)
% AND if Task Program actually supplies appropriate feedback styles (size(VCODES_in,2)==70)
if fdbk_src_GUI==0 && block_settings==3 && size(VCODES_in,2)==70
    VCODES=VCODES_in;
else
    VCODES=zeros(2,70);						%set default
	VCODES(:,1)=1;							%target_type of circle
	VCODES(:,5)=fdbk_clr_GUI;				%fill colour as specified by GUI
	VCODES(:,6)=fdbk_clr_GUI;				%stroke colour same as fill colour
	VCODES(:,7)=0;							%no stroke width
    VCODES(:,9)=100.0;                      %100% opacity
	VCODES(:,10)=fdbk_radius_GUI;			%radius (m) as specified by GUI
end

%----------------Feedback Status ----------------
%feedback status from GUI sets the default to be used
feedback_status=fdbk_stts_GUI;


if fdbk_stts_GUI==4				%if GUI has requested Task Program control of feedback status
	if block_settings==2		%if there is Task Program control ONLY of status (but not style)
		feedback_status=fdbk_stts_mdl;		%then use feedback status input from parent block
	elseif block_settings==3	%if there is Task Program control of both status and style
		feedback_status=4;		%then let the input VCODEs handle the status
	else						%otherwise assume that the Task Program did not provide style OR status
		feedback_status=3;		%then set both hands are always on as a default
    end
else		%if GUI is controlling feedback status
	feedback_status=fdbk_stts_GUI;
end

%set the status of the hand-feedback in the VCODES
switch feedback_status
	case 0					%show neither hand feedback
		VCODES(1,2)=0;
		VCODES(2,2)=0;
	case 1					%show ONLY dominant hand feedback
		VCODES(1,2)=1;
		VCODES(2,2)=0;
	case 2					%show ONLY non-dominant hand feedback
		VCODES(1,2)=0;
		VCODES(2,2)=1;
	case 4					%VCODES already control hand feedback
		%do nothing
	otherwise				%show both hand feedbacks
		VCODES(1,2)=1;
		VCODES(2,2)=1;
end

%----------------Feedback Position ----------------
%set the position of the hand feedback.
for i=1:2
	if i==1
		active_arm=KINARMdata(3,1);			%choose dominant arm first
	else
		active_arm=3-KINARMdata(3,1);		%choose non-dominant arm 2nd
	end
	HandXPos=KINARMdata(active_arm,23);		%(m)
	HandYPos=KINARMdata(active_arm,24);		%(m)
	HandXVel=KINARMdata(active_arm,25);		%(m/s)
	HandYVel=KINARMdata(active_arm,26);		%(m/s)

	% feed-forward hand position (m)
	%HandXPos_ff = HandXPos + HandXVel*feedfwd;
	%HandYPos_ff = HandYPos + HandYVel*feedfwd;
	HandXPos_ff = HandXPos;
	HandYPos_ff = HandYPos;
	VCODES(i,3)=HandXPos_ff;				%target position in m 
	VCODES(i,4)=HandYPos_ff;				%target position in m 
end

VCODES_out=VCODES;
